simulink model "assignment1"  (R2023b)
settings: Solver=FixedStepAuto  StartTime=0.0  StopTime=10.0  FixedStep=1e-3  RelTol=1e-3  EnableMultiTasking=on
undefined symbols (not defined in the file): D0, D1, PTC16, PTC17
libraries: frdmk64flib x2
settings Model: ExtModeTrigDuration=5  Creator=jesti  LastModifiedBy=jesti
settings OptimizationCC: EnhancedBackFolding=on  PassReuseOutputArgsAs=Individual arguments  ZeroExternalMemoryAtStartup=off  ZeroInternalMemoryAtStartup=off  MaxStackSize=64  OptimizeBlockOrder=speed  DifferentSizesBufferReuse=on  OptimizationCustomize=off  EfficientTunableParamExpr=on
settings DebuggingCC: ParameterTunabilityLossMsg=error
settings HardwareCC: ProdBitPerPointer=32  ProdBitPerSizeT=32  ProdBitPerPtrDiffT=32  ProdLargestAtomicInteger=Long  ProdLargestAtomicFloat=Double  ProdWordSize=32  ProdHWDeviceType=ARM Compatible->ARM Cortex
settings SFSimCC: MATLABDynamicMemAlloc=off
settings RTWCC: Description=Embedded Coder  SystemTargetFile=ert.tlc  HardwareBoard=NXP FRDM-K64F  TLCOptions="-aInlineSetEventsForThisBaseRateFcn=TLC_FALSE -aSuppressMultiTaskScheduler=TLC_FALSE  -aRateBasedStepFcn=0"  TemplateMakefile=ert_default_tmf  Toolchain=GNU Tools for ARM Embedded Processors
settings CodeAppCC: ForceParamTrailComments=on  IgnoreCustomStorageClasses=off  OperatorAnnotations=on  SimulinkDataObjDesc=on  SFDataObjDesc=on  InsertBlockDesc=on
settings ERTTargetCC: ExtModeTransport=4  ExtModeMexFile=sendToCommService

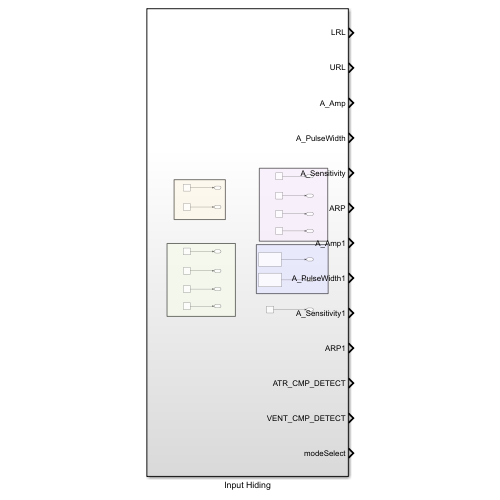
[thumbnail: Simulink's stored preview of the top-level diagram]
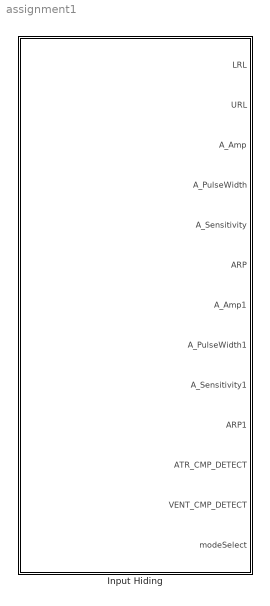
== system assignment1 ==
  Input Hiding : Subsystem

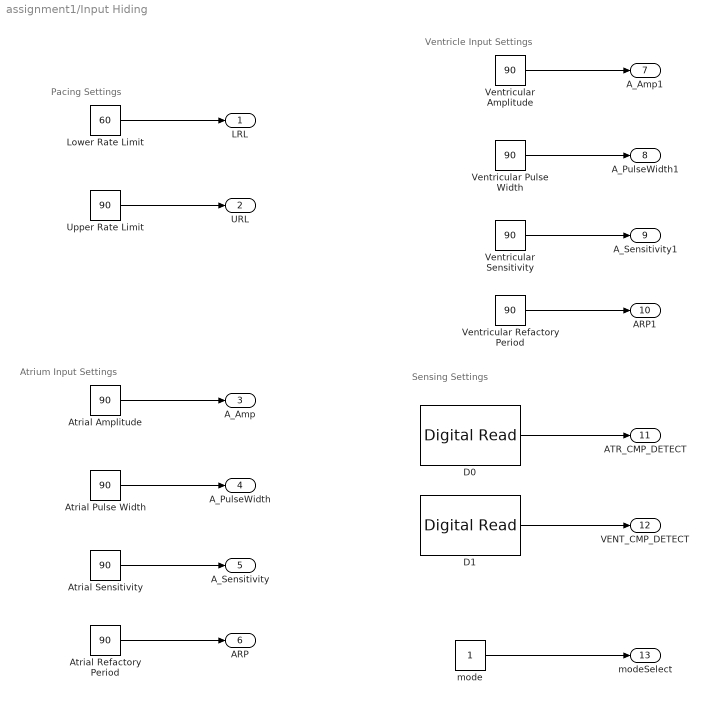
== system assignment1/Input Hiding ==
  note: Sensing Settings
  note: Pacing Settings
  note: Atrium Input Settings
  note: Ventricle Input Settings
  "Atrial Amplitude " : Constant  Value=90  OutDataTypeStr=double
  Atrial Pulse Width : Constant  Value=90  OutDataTypeStr=double
  Atrial Refactory Period : Constant  Value=90  OutDataTypeStr=double
  Atrial Sensitivity : Constant  Value=90  OutDataTypeStr=double
  D0 : frdmk64flib/Digital Read  Whichpin=PTC16 (D0)  SampleTime=-1
  D1 : frdmk64flib/Digital Read  Whichpin=PTC17 (D1)  SampleTime=-1
  Lower Rate Limit : Constant  Value=60  OutDataTypeStr=double
  Upper Rate Limit : Constant  Value=90  OutDataTypeStr=double
  Ventricular Amplitude : Constant  Value=90  OutDataTypeStr=double
  Ventricular Pulse Width : Constant  Value=90  OutDataTypeStr=double
  Ventricular Refactory Period : Constant  Value=90  OutDataTypeStr=double
  Ventricular Sensitivity : Constant  Value=90  OutDataTypeStr=double
  mode : Constant
  LRL : Outport  OutDataTypeStr=double
  URL : Outport  Port=2  OutDataTypeStr=double
  A_Amp : Outport  Port=3  OutDataTypeStr=double
  A_PulseWidth : Outport  Port=4  OutDataTypeStr=double
  A_Sensitivity : Outport  Port=5  OutDataTypeStr=double
  ARP : Outport  Port=6  OutDataTypeStr=double
  A_Amp1 : Outport  Port=7  OutDataTypeStr=double
  A_PulseWidth1 : Outport  Port=8  OutDataTypeStr=double
  A_Sensitivity1 : Outport  Port=9  OutDataTypeStr=double
  ARP1 : Outport  Port=10  OutDataTypeStr=double
  ATR_CMP_DETECT : Outport  Port=11  OutDataTypeStr=boolean
  VENT_CMP_DETECT : Outport  Port=12  OutDataTypeStr=boolean
  modeSelect : Outport  Port=13
  wires:
  Lower Rate Limit/1 -> LRL/1
  Upper Rate Limit/1 -> URL/1
  "Atrial Amplitude "/1 -> A_Amp/1
  Atrial Pulse Width/1 -> A_PulseWidth/1
  Atrial Sensitivity/1 -> A_Sensitivity/1
  Atrial Refactory Period/1 -> ARP/1
  Ventricular Refactory Period/1 -> ARP1/1
  Ventricular Sensitivity/1 -> A_Sensitivity1/1
  Ventricular Amplitude/1 -> A_Amp1/1
  Ventricular Pulse Width/1 -> A_PulseWidth1/1
  D1/1 -> VENT_CMP_DETECT/1
  D0/1 -> ATR_CMP_DETECT/1
  mode/1 -> modeSelect/1
